simulink model "MPU6050_real_time"  (R2023a)
settings: Solver=FixedStepAuto  StartTime=0.0  StopTime=10  RelTol=1e-3
libraries: arduinosensorlib x2
settings Model: ExtModeTrigDuration=2  Creator=admin  LastModifiedBy=admin
settings OptimizationCC: EnhancedBackFolding=on  PassReuseOutputArgsAs=Individual arguments  ZeroExternalMemoryAtStartup=off  ZeroInternalMemoryAtStartup=off  MaxStackSize=64  OptimizeBlockOrder=speed  DifferentSizesBufferReuse=on  OptimizationCustomize=off  EfficientTunableParamExpr=on
settings DebuggingCC: ParameterTunabilityLossMsg=error
settings HardwareCC: ProdBitPerInt=16  ProdBitPerPointer=16  ProdBitPerSizeT=16  ProdBitPerPtrDiffT=16  ProdLargestAtomicFloat=None  ProdWordSize=8  ProdHWDeviceType=Atmel->AVR
settings SFSimCC: MATLABDynamicMemAlloc=off
settings RTWCC: Description=Embedded Coder  SystemTargetFile=ert.tlc  HardwareBoard=Arduino Uno  TemplateMakefile=ert_default_tmf  Toolchain=Arduino AVR
settings CodeAppCC: ForceParamTrailComments=on  IgnoreCustomStorageClasses=off  OperatorAnnotations=on  SimulinkDataObjDesc=on  SFDataObjDesc=on  InsertBlockDesc=on
settings ERTTargetCC: SupportContinuousTime=on  SupportVariableSizeSignals=on  ExtModeTransport=3  ExtModeStaticAlloc=on  ExtModeAutomaticAllocSize=off  ExtModeStaticAllocSize=250  ExtModeMexFile=ext_xcp  ExtModeIntrfLevel=Level2 - Open

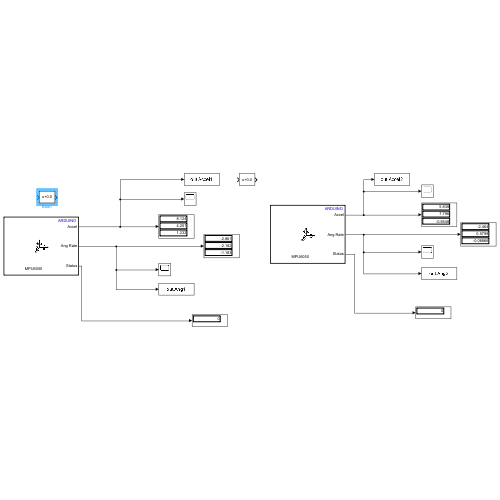
[thumbnail: Simulink's stored preview of the top-level diagram]
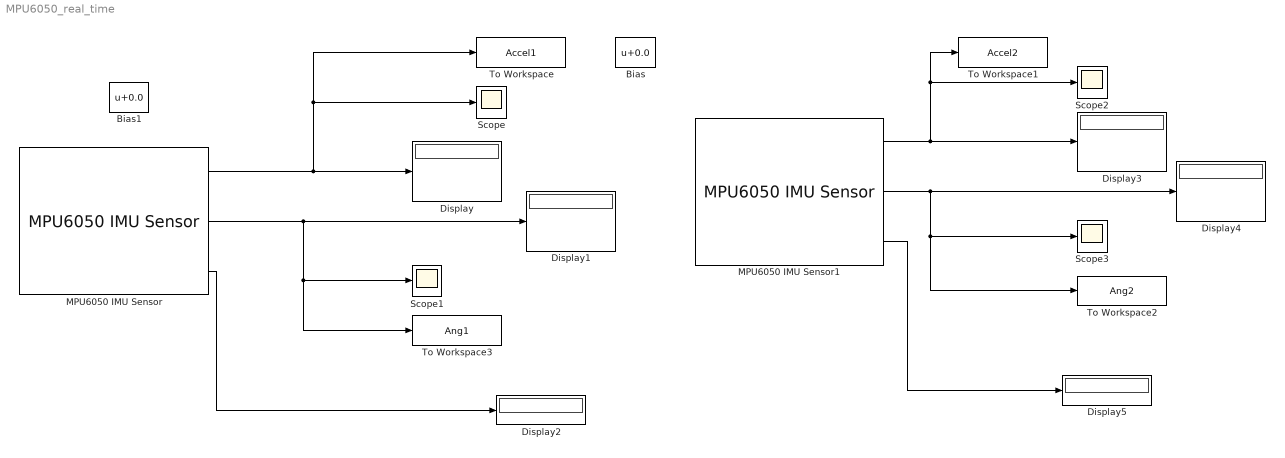
== system MPU6050_real_time ==
  Bias : Bias  Bias=0.0  SaturateOnIntegerOverflow=off
  Bias1 : Bias  Bias=0.0  SaturateOnIntegerOverflow=off
  Display{,1..5} (6 alike) : Display
  MPU6050 IMU Sensor : arduinosensorlib/MPU6050 IMU Sensor  SlaveAddress=0x68  Accel=on  AngularRate=on  Temperature=off  Status=on  Timestamp=off  EulerAngles=off  Quat=off  AccelRange=2G  GyroRange=250 dps  DmpOdr=200 Hz  Dlpf=Accelerometer: 184Hz, Gyroscope: 188Hz  spf=1  SampleTime=0.01  QueueSizeFactor=1
  MPU6050 IMU Sensor1 : arduinosensorlib/MPU6050 IMU Sensor  SlaveAddress=0x69  Accel=on  AngularRate=on  Temperature=off  Status=on  Timestamp=off  EulerAngles=off  Quat=off  AccelRange=2G  GyroRange=250 dps  DmpOdr=200 Hz  Dlpf=Accelerometer: 184Hz, Gyroscope: 188Hz  spf=1  SampleTime=0.01  QueueSizeFactor=1
  Scope{,1..3} (4 alike) : Scope
  To Workspace : ToWorkspace  VariableName=Accel1  SaveFormat=Timeseries  SampleTime=-1
  To Workspace1 : ToWorkspace  VariableName=Accel2  SaveFormat=Timeseries  SampleTime=-1
  To Workspace2 : ToWorkspace  VariableName=Ang2  SaveFormat=Timeseries  SampleTime=-1
  To Workspace3 : ToWorkspace  VariableName=Ang1  SaveFormat=Timeseries  SampleTime=-1
  wires:
  MPU6050 IMU Sensor/3 -> Display2/1
  MPU6050 IMU Sensor/2 -> Display1/1, To Workspace3/1, Scope1/1
  MPU6050 IMU Sensor1/1 -> Scope2/1, To Workspace1/1, Display3/1
  MPU6050 IMU Sensor1/3 -> Display5/1
  MPU6050 IMU Sensor1/2 -> To Workspace2/1, Scope3/1, Display4/1
  MPU6050 IMU Sensor/1 -> Display/1, Scope/1, To Workspace/1
